simulink model "Snake_Robot_v1"  (R2022b)
settings: Solver=VariableStepAuto  StartTime=0.0  StopTime=300  RelTol=1e-5  AbsTol=1e-3  EnableMultiTasking=on
values from neighbouring files (symbols this model uses):
  amplitude = 2.5    [Snake_robot_parameters.m]
  frequency = 2    [Snake_robot_parameters.m]
  lookup_table_x = [-3 -1.5 -1 1 1.5 3]    [Snake_robot_parameters.m]
  lookup_table_y = [-3 -1.5 -1 1 1.5 3]    [Snake_robot_parameters.m]
  muk_x = 1e-5    (= 1e-05)    [Snake_robot_parameters.m]
  muk_y = 10    [Snake_robot_parameters.m]
  mus_x = 1e-4    (= 0.0001)    [Snake_robot_parameters.m]
  mus_y = 13    [Snake_robot_parameters.m]
  phase = 1.4    [Snake_robot_parameters.m]
undefined symbols (not defined in the file or in its folder): X, Y, Z
libraries: nesl_utility x88, sm_lib x74, simulink x53, slpidlib x5, robotalgslib x1
(part 3 of 4)

== system Snake_Robot_v1/body_1/custom friction law2 ==
  Demux : Demux  Outputs=2
  PS-Simulink Converter1 : nesl_utility/PS-Simulink Converter  PhysicalDomain=network_engine_domain  SubClassName=ps_output  LeftPortType=input  RightPortType=output  PseudoPeriodic=off  Frequencies=[]  VectorFormat=inherit  Unit=inherit  AffineConversion=off
  PS-Simulink Converter4 : nesl_utility/PS-Simulink Converter  PhysicalDomain=network_engine_domain  SubClassName=ps_output  LeftPortType=input  RightPortType=output  PseudoPeriodic=off  Frequencies=[]  VectorFormat=inherit  Unit=inherit  AffineConversion=off
  Scope{,1..3} (4 alike) : Scope
  Simulink-PS Converter : nesl_utility/Simulink-PS Converter  PhysicalDomain=network_engine_domain  SubClassName=ps_input  LeftPortType=input  RightPortType=output  PseudoPeriodic=off  Frequencies=[]  NoiseDistribution=none  NoiseParameters=[]  Unit=1  AffineConversion=off  FilteringAndDerivatives=provide  SimscapeFilterOrder=1  InputFilterTimeConstant=0.001  UdotUserProvided=0
  Spatial Contact Force : sm_lib/Forces and Torques/Spatial Contact Force  SenseContactBaseRotation=off  SenseContactBaseTranslation=off  CoefficientOfDynamicFriction=mu_dynamic  CoefficientOfStaticFriction=mu_static  NormalDamping=1e3  NormalDampingUnits=N/(m/s)  SenseContactSignal=off  NormalStiffness=1e6  NormalStiffnessUnits=N/m  FrictionalCriticalVelocity=1e-3  FrictionalCriticalVelocityUnits=m/s  ZeroCrossDetectContactStartAndEnd=off  SenseContactFollowerRotation=off  SenseContactFollowerTranslation=off  FrictionType=ProvidedByInput  SenseFrictionalForceMagnitude=off  SenseNormalForceMagnitude=on  NormalForceType=SmoothSpringDamper  SenseNormalVelocity=off  SenseSeparationDistance=off  SenseTangentialVelocity=on  NormalTransitionRegionWidth=1e-4  NormalTransitionRegionWidthUnits=m
  custom friction law : Subsystem
  body : PMIOPort  Side=Right
  ground : PMIOPort  Port=2  Side=Left
  wires:
  PS-Simulink Converter1/1 -> Demux/1, custom friction law/2(velocity)  "velocity"
  PS-Simulink Converter4/1 -> Scope1/1, custom friction law/1(normal force)  "normal force"
  custom friction law/1(Friction force) -> Scope/1, Simulink-PS Converter/1  "friction force"
  Demux/1 -> Scope2/1
  Demux/2 -> Scope3/1
  connections:
  Spatial Contact Force/LConn1 -- ground/RConn1
  Spatial Contact Force/RConn2 -- PS-Simulink Converter4/LConn1
  Simulink-PS Converter/RConn1 -- Spatial Contact Force/LConn2
  Spatial Contact Force/RConn3 -- PS-Simulink Converter1/LConn1
  Spatial Contact Force/RConn1 -- body/RConn1

== system Snake_Robot_v1/body_1/custom friction law3 ==
  Demux : Demux  Outputs=2
  PS-Simulink Converter1 : nesl_utility/PS-Simulink Converter  PhysicalDomain=network_engine_domain  SubClassName=ps_output  LeftPortType=input  RightPortType=output  PseudoPeriodic=off  Frequencies=[]  VectorFormat=inherit  Unit=inherit  AffineConversion=off
  PS-Simulink Converter4 : nesl_utility/PS-Simulink Converter  PhysicalDomain=network_engine_domain  SubClassName=ps_output  LeftPortType=input  RightPortType=output  PseudoPeriodic=off  Frequencies=[]  VectorFormat=inherit  Unit=inherit  AffineConversion=off
  Scope{,1..3} (4 alike) : Scope
  Simulink-PS Converter : nesl_utility/Simulink-PS Converter  PhysicalDomain=network_engine_domain  SubClassName=ps_input  LeftPortType=input  RightPortType=output  PseudoPeriodic=off  Frequencies=[]  NoiseDistribution=none  NoiseParameters=[]  Unit=1  AffineConversion=off  FilteringAndDerivatives=provide  SimscapeFilterOrder=1  InputFilterTimeConstant=0.001  UdotUserProvided=0
  Spatial Contact Force : sm_lib/Forces and Torques/Spatial Contact Force  SenseContactBaseRotation=off  SenseContactBaseTranslation=off  CoefficientOfDynamicFriction=mu_dynamic  CoefficientOfStaticFriction=mu_static  NormalDamping=1e3  NormalDampingUnits=N/(m/s)  SenseContactSignal=off  NormalStiffness=1e6  NormalStiffnessUnits=N/m  FrictionalCriticalVelocity=1e-3  FrictionalCriticalVelocityUnits=m/s  ZeroCrossDetectContactStartAndEnd=off  SenseContactFollowerRotation=off  SenseContactFollowerTranslation=off  FrictionType=ProvidedByInput  SenseFrictionalForceMagnitude=off  SenseNormalForceMagnitude=on  NormalForceType=SmoothSpringDamper  SenseNormalVelocity=off  SenseSeparationDistance=off  SenseTangentialVelocity=on  NormalTransitionRegionWidth=1e-4  NormalTransitionRegionWidthUnits=m
  custom friction law : Subsystem
  body : PMIOPort  Side=Right
  ground : PMIOPort  Port=2  Side=Left
  wires:
  Demux/2 -> Scope3/1
  Demux/1 -> Scope2/1
  custom friction law/1(Friction force) -> Simulink-PS Converter/1, Scope/1  "friction force"
  PS-Simulink Converter4/1 -> custom friction law/1(normal force), Scope1/1  "normal force"
  PS-Simulink Converter1/1 -> custom friction law/2(velocity), Demux/1  "velocity"
  connections:
  Spatial Contact Force/RConn1 -- body/RConn1
  Spatial Contact Force/RConn3 -- PS-Simulink Converter1/LConn1
  Simulink-PS Converter/RConn1 -- Spatial Contact Force/LConn2
  Spatial Contact Force/RConn2 -- PS-Simulink Converter4/LConn1
  Spatial Contact Force/LConn1 -- ground/RConn1

== system Snake_Robot_v1/body_2/custom friction law ==
  Demux : Demux  Outputs=2
  PS-Simulink Converter1 : nesl_utility/PS-Simulink Converter  PhysicalDomain=network_engine_domain  SubClassName=ps_output  LeftPortType=input  RightPortType=output  PseudoPeriodic=off  Frequencies=[]  VectorFormat=inherit  Unit=inherit  AffineConversion=off
  PS-Simulink Converter4 : nesl_utility/PS-Simulink Converter  PhysicalDomain=network_engine_domain  SubClassName=ps_output  LeftPortType=input  RightPortType=output  PseudoPeriodic=off  Frequencies=[]  VectorFormat=inherit  Unit=inherit  AffineConversion=off
  Scope{,1..3} (4 alike) : Scope
  Simulink-PS Converter : nesl_utility/Simulink-PS Converter  PhysicalDomain=network_engine_domain  SubClassName=ps_input  LeftPortType=input  RightPortType=output  PseudoPeriodic=off  Frequencies=[]  NoiseDistribution=none  NoiseParameters=[]  Unit=1  AffineConversion=off  FilteringAndDerivatives=provide  SimscapeFilterOrder=1  InputFilterTimeConstant=0.001  UdotUserProvided=0
  Spatial Contact Force : sm_lib/Forces and Torques/Spatial Contact Force  SenseContactBaseRotation=off  SenseContactBaseTranslation=off  CoefficientOfDynamicFriction=mu_dynamic  CoefficientOfStaticFriction=mu_static  NormalDamping=1e3  NormalDampingUnits=N/(m/s)  SenseContactSignal=off  NormalStiffness=1e6  NormalStiffnessUnits=N/m  FrictionalCriticalVelocity=1e-3  FrictionalCriticalVelocityUnits=m/s  ZeroCrossDetectContactStartAndEnd=off  SenseContactFollowerRotation=off  SenseContactFollowerTranslation=off  FrictionType=ProvidedByInput  SenseFrictionalForceMagnitude=off  SenseNormalForceMagnitude=on  NormalForceType=SmoothSpringDamper  SenseNormalVelocity=off  SenseSeparationDistance=off  SenseTangentialVelocity=on  NormalTransitionRegionWidth=1e-4  NormalTransitionRegionWidthUnits=m
  custom friction law : Subsystem
  body : PMIOPort  Side=Right
  ground : PMIOPort  Port=2  Side=Left
  wires:
  Demux/2 -> Scope3/1
  Demux/1 -> Scope2/1
  custom friction law/1(Friction force) -> Simulink-PS Converter/1, Scope/1  "friction force"
  PS-Simulink Converter4/1 -> custom friction law/1(normal force), Scope1/1  "normal force"
  PS-Simulink Converter1/1 -> custom friction law/2(velocity), Demux/1  "velocity"
  connections:
  Spatial Contact Force/RConn1 -- body/RConn1
  Spatial Contact Force/RConn3 -- PS-Simulink Converter1/LConn1
  Simulink-PS Converter/RConn1 -- Spatial Contact Force/LConn2
  Spatial Contact Force/RConn2 -- PS-Simulink Converter4/LConn1
  Spatial Contact Force/LConn1 -- ground/RConn1

== system Snake_Robot_v1/body_2/custom friction law1 ==
  Demux : Demux  Outputs=2
  PS-Simulink Converter1 : nesl_utility/PS-Simulink Converter  PhysicalDomain=network_engine_domain  SubClassName=ps_output  LeftPortType=input  RightPortType=output  PseudoPeriodic=off  Frequencies=[]  VectorFormat=inherit  Unit=inherit  AffineConversion=off
  PS-Simulink Converter4 : nesl_utility/PS-Simulink Converter  PhysicalDomain=network_engine_domain  SubClassName=ps_output  LeftPortType=input  RightPortType=output  PseudoPeriodic=off  Frequencies=[]  VectorFormat=inherit  Unit=inherit  AffineConversion=off
  Scope{,1..3} (4 alike) : Scope
  Simulink-PS Converter : nesl_utility/Simulink-PS Converter  PhysicalDomain=network_engine_domain  SubClassName=ps_input  LeftPortType=input  RightPortType=output  PseudoPeriodic=off  Frequencies=[]  NoiseDistribution=none  NoiseParameters=[]  Unit=1  AffineConversion=off  FilteringAndDerivatives=provide  SimscapeFilterOrder=1  InputFilterTimeConstant=0.001  UdotUserProvided=0
  Spatial Contact Force : sm_lib/Forces and Torques/Spatial Contact Force  SenseContactBaseRotation=off  SenseContactBaseTranslation=off  CoefficientOfDynamicFriction=mu_dynamic  CoefficientOfStaticFriction=mu_static  NormalDamping=1e3  NormalDampingUnits=N/(m/s)  SenseContactSignal=off  NormalStiffness=1e6  NormalStiffnessUnits=N/m  FrictionalCriticalVelocity=1e-3  FrictionalCriticalVelocityUnits=m/s  ZeroCrossDetectContactStartAndEnd=off  SenseContactFollowerRotation=off  SenseContactFollowerTranslation=off  FrictionType=ProvidedByInput  SenseFrictionalForceMagnitude=off  SenseNormalForceMagnitude=on  NormalForceType=SmoothSpringDamper  SenseNormalVelocity=off  SenseSeparationDistance=off  SenseTangentialVelocity=on  NormalTransitionRegionWidth=1e-4  NormalTransitionRegionWidthUnits=m
  custom friction law : Subsystem
  body : PMIOPort  Side=Right
  ground : PMIOPort  Port=2  Side=Left
  wires:
  PS-Simulink Converter1/1 -> Demux/1, custom friction law/2(velocity)  "velocity"
  PS-Simulink Converter4/1 -> Scope1/1, custom friction law/1(normal force)  "normal force"
  custom friction law/1(Friction force) -> Scope/1, Simulink-PS Converter/1  "friction force"
  Demux/1 -> Scope2/1
  Demux/2 -> Scope3/1
  connections:
  Spatial Contact Force/LConn1 -- ground/RConn1
  Spatial Contact Force/RConn2 -- PS-Simulink Converter4/LConn1
  Simulink-PS Converter/RConn1 -- Spatial Contact Force/LConn2
  Spatial Contact Force/RConn3 -- PS-Simulink Converter1/LConn1
  Spatial Contact Force/RConn1 -- body/RConn1

== system Snake_Robot_v1/body_2/custom friction law2 ==
  Demux : Demux  Outputs=2
  PS-Simulink Converter1 : nesl_utility/PS-Simulink Converter  PhysicalDomain=network_engine_domain  SubClassName=ps_output  LeftPortType=input  RightPortType=output  PseudoPeriodic=off  Frequencies=[]  VectorFormat=inherit  Unit=inherit  AffineConversion=off
  PS-Simulink Converter4 : nesl_utility/PS-Simulink Converter  PhysicalDomain=network_engine_domain  SubClassName=ps_output  LeftPortType=input  RightPortType=output  PseudoPeriodic=off  Frequencies=[]  VectorFormat=inherit  Unit=inherit  AffineConversion=off
  Scope{,1..3} (4 alike) : Scope
  Simulink-PS Converter : nesl_utility/Simulink-PS Converter  PhysicalDomain=network_engine_domain  SubClassName=ps_input  LeftPortType=input  RightPortType=output  PseudoPeriodic=off  Frequencies=[]  NoiseDistribution=none  NoiseParameters=[]  Unit=1  AffineConversion=off  FilteringAndDerivatives=provide  SimscapeFilterOrder=1  InputFilterTimeConstant=0.001  UdotUserProvided=0
  Spatial Contact Force : sm_lib/Forces and Torques/Spatial Contact Force  SenseContactBaseRotation=off  SenseContactBaseTranslation=off  CoefficientOfDynamicFriction=mu_dynamic  CoefficientOfStaticFriction=mu_static  NormalDamping=1e3  NormalDampingUnits=N/(m/s)  SenseContactSignal=off  NormalStiffness=1e6  NormalStiffnessUnits=N/m  FrictionalCriticalVelocity=1e-3  FrictionalCriticalVelocityUnits=m/s  ZeroCrossDetectContactStartAndEnd=off  SenseContactFollowerRotation=off  SenseContactFollowerTranslation=off  FrictionType=ProvidedByInput  SenseFrictionalForceMagnitude=off  SenseNormalForceMagnitude=on  NormalForceType=SmoothSpringDamper  SenseNormalVelocity=off  SenseSeparationDistance=off  SenseTangentialVelocity=on  NormalTransitionRegionWidth=1e-4  NormalTransitionRegionWidthUnits=m
  custom friction law : Subsystem
  body : PMIOPort  Side=Right
  ground : PMIOPort  Port=2  Side=Left
  wires:
  Demux/2 -> Scope3/1
  Demux/1 -> Scope2/1
  custom friction law/1(Friction force) -> Simulink-PS Converter/1, Scope/1  "friction force"
  PS-Simulink Converter4/1 -> custom friction law/1(normal force), Scope1/1  "normal force"
  PS-Simulink Converter1/1 -> custom friction law/2(velocity), Demux/1  "velocity"
  connections:
  Spatial Contact Force/RConn1 -- body/RConn1
  Spatial Contact Force/RConn3 -- PS-Simulink Converter1/LConn1
  Simulink-PS Converter/RConn1 -- Spatial Contact Force/LConn2
  Spatial Contact Force/RConn2 -- PS-Simulink Converter4/LConn1
  Spatial Contact Force/LConn1 -- ground/RConn1

== system Snake_Robot_v1/body_2/custom friction law3 ==
  Demux : Demux  Outputs=2
  PS-Simulink Converter1 : nesl_utility/PS-Simulink Converter  PhysicalDomain=network_engine_domain  SubClassName=ps_output  LeftPortType=input  RightPortType=output  PseudoPeriodic=off  Frequencies=[]  VectorFormat=inherit  Unit=inherit  AffineConversion=off
  PS-Simulink Converter4 : nesl_utility/PS-Simulink Converter  PhysicalDomain=network_engine_domain  SubClassName=ps_output  LeftPortType=input  RightPortType=output  PseudoPeriodic=off  Frequencies=[]  VectorFormat=inherit  Unit=inherit  AffineConversion=off
  Scope{,1..3} (4 alike) : Scope
  Simulink-PS Converter : nesl_utility/Simulink-PS Converter  PhysicalDomain=network_engine_domain  SubClassName=ps_input  LeftPortType=input  RightPortType=output  PseudoPeriodic=off  Frequencies=[]  NoiseDistribution=none  NoiseParameters=[]  Unit=1  AffineConversion=off  FilteringAndDerivatives=provide  SimscapeFilterOrder=1  InputFilterTimeConstant=0.001  UdotUserProvided=0
  Spatial Contact Force : sm_lib/Forces and Torques/Spatial Contact Force  SenseContactBaseRotation=off  SenseContactBaseTranslation=off  CoefficientOfDynamicFriction=mu_dynamic  CoefficientOfStaticFriction=mu_static  NormalDamping=1e3  NormalDampingUnits=N/(m/s)  SenseContactSignal=off  NormalStiffness=1e6  NormalStiffnessUnits=N/m  FrictionalCriticalVelocity=1e-3  FrictionalCriticalVelocityUnits=m/s  ZeroCrossDetectContactStartAndEnd=off  SenseContactFollowerRotation=off  SenseContactFollowerTranslation=off  FrictionType=ProvidedByInput  SenseFrictionalForceMagnitude=off  SenseNormalForceMagnitude=on  NormalForceType=SmoothSpringDamper  SenseNormalVelocity=off  SenseSeparationDistance=off  SenseTangentialVelocity=on  NormalTransitionRegionWidth=1e-4  NormalTransitionRegionWidthUnits=m
  custom friction law : Subsystem
  body : PMIOPort  Side=Right
  ground : PMIOPort  Port=2  Side=Left
  wires:
  PS-Simulink Converter1/1 -> Demux/1, custom friction law/2(velocity)  "velocity"
  PS-Simulink Converter4/1 -> Scope1/1, custom friction law/1(normal force)  "normal force"
  custom friction law/1(Friction force) -> Scope/1, Simulink-PS Converter/1  "friction force"
  Demux/1 -> Scope2/1
  Demux/2 -> Scope3/1
  connections:
  Spatial Contact Force/LConn1 -- ground/RConn1
  Spatial Contact Force/RConn2 -- PS-Simulink Converter4/LConn1
  Simulink-PS Converter/RConn1 -- Spatial Contact Force/LConn2
  Spatial Contact Force/RConn3 -- PS-Simulink Converter1/LConn1
  Spatial Contact Force/RConn1 -- body/RConn1

== system Snake_Robot_v1/body_3/custom friction law ==
  Demux : Demux  Outputs=2
  PS-Simulink Converter1 : nesl_utility/PS-Simulink Converter  PhysicalDomain=network_engine_domain  SubClassName=ps_output  LeftPortType=input  RightPortType=output  PseudoPeriodic=off  Frequencies=[]  VectorFormat=inherit  Unit=inherit  AffineConversion=off
  PS-Simulink Converter4 : nesl_utility/PS-Simulink Converter  PhysicalDomain=network_engine_domain  SubClassName=ps_output  LeftPortType=input  RightPortType=output  PseudoPeriodic=off  Frequencies=[]  VectorFormat=inherit  Unit=inherit  AffineConversion=off
  Scope{,1..3} (4 alike) : Scope
  Simulink-PS Converter : nesl_utility/Simulink-PS Converter  PhysicalDomain=network_engine_domain  SubClassName=ps_input  LeftPortType=input  RightPortType=output  PseudoPeriodic=off  Frequencies=[]  NoiseDistribution=none  NoiseParameters=[]  Unit=1  AffineConversion=off  FilteringAndDerivatives=provide  SimscapeFilterOrder=1  InputFilterTimeConstant=0.001  UdotUserProvided=0
  Spatial Contact Force : sm_lib/Forces and Torques/Spatial Contact Force  SenseContactBaseRotation=off  SenseContactBaseTranslation=off  CoefficientOfDynamicFriction=mu_dynamic  CoefficientOfStaticFriction=mu_static  NormalDamping=1e3  NormalDampingUnits=N/(m/s)  SenseContactSignal=off  NormalStiffness=1e6  NormalStiffnessUnits=N/m  FrictionalCriticalVelocity=1e-3  FrictionalCriticalVelocityUnits=m/s  ZeroCrossDetectContactStartAndEnd=off  SenseContactFollowerRotation=off  SenseContactFollowerTranslation=off  FrictionType=ProvidedByInput  SenseFrictionalForceMagnitude=off  SenseNormalForceMagnitude=on  NormalForceType=SmoothSpringDamper  SenseNormalVelocity=off  SenseSeparationDistance=off  SenseTangentialVelocity=on  NormalTransitionRegionWidth=1e-4  NormalTransitionRegionWidthUnits=m
  custom friction law : Subsystem
  body : PMIOPort  Side=Right
  ground : PMIOPort  Port=2  Side=Left
  wires:
  PS-Simulink Converter1/1 -> Demux/1, custom friction law/2(velocity)  "velocity"
  PS-Simulink Converter4/1 -> Scope1/1, custom friction law/1(normal force)  "normal force"
  custom friction law/1(Friction force) -> Scope/1, Simulink-PS Converter/1  "friction force"
  Demux/1 -> Scope2/1
  Demux/2 -> Scope3/1
  connections:
  Spatial Contact Force/LConn1 -- ground/RConn1
  Spatial Contact Force/RConn2 -- PS-Simulink Converter4/LConn1
  Simulink-PS Converter/RConn1 -- Spatial Contact Force/LConn2
  Spatial Contact Force/RConn3 -- PS-Simulink Converter1/LConn1
  Spatial Contact Force/RConn1 -- body/RConn1

== system Snake_Robot_v1/body_3/custom friction law1 ==
  Demux : Demux  Outputs=2
  PS-Simulink Converter1 : nesl_utility/PS-Simulink Converter  PhysicalDomain=network_engine_domain  SubClassName=ps_output  LeftPortType=input  RightPortType=output  PseudoPeriodic=off  Frequencies=[]  VectorFormat=inherit  Unit=inherit  AffineConversion=off
  PS-Simulink Converter4 : nesl_utility/PS-Simulink Converter  PhysicalDomain=network_engine_domain  SubClassName=ps_output  LeftPortType=input  RightPortType=output  PseudoPeriodic=off  Frequencies=[]  VectorFormat=inherit  Unit=inherit  AffineConversion=off
  Scope{,1..3} (4 alike) : Scope
  Simulink-PS Converter : nesl_utility/Simulink-PS Converter  PhysicalDomain=network_engine_domain  SubClassName=ps_input  LeftPortType=input  RightPortType=output  PseudoPeriodic=off  Frequencies=[]  NoiseDistribution=none  NoiseParameters=[]  Unit=1  AffineConversion=off  FilteringAndDerivatives=provide  SimscapeFilterOrder=1  InputFilterTimeConstant=0.001  UdotUserProvided=0
  Spatial Contact Force : sm_lib/Forces and Torques/Spatial Contact Force  SenseContactBaseRotation=off  SenseContactBaseTranslation=off  CoefficientOfDynamicFriction=mu_dynamic  CoefficientOfStaticFriction=mu_static  NormalDamping=1e3  NormalDampingUnits=N/(m/s)  SenseContactSignal=off  NormalStiffness=1e6  NormalStiffnessUnits=N/m  FrictionalCriticalVelocity=1e-3  FrictionalCriticalVelocityUnits=m/s  ZeroCrossDetectContactStartAndEnd=off  SenseContactFollowerRotation=off  SenseContactFollowerTranslation=off  FrictionType=ProvidedByInput  SenseFrictionalForceMagnitude=off  SenseNormalForceMagnitude=on  NormalForceType=SmoothSpringDamper  SenseNormalVelocity=off  SenseSeparationDistance=off  SenseTangentialVelocity=on  NormalTransitionRegionWidth=1e-4  NormalTransitionRegionWidthUnits=m
  custom friction law : Subsystem
  body : PMIOPort  Side=Right
  ground : PMIOPort  Port=2  Side=Left
  wires:
  Demux/2 -> Scope3/1
  Demux/1 -> Scope2/1
  custom friction law/1(Friction force) -> Simulink-PS Converter/1, Scope/1  "friction force"
  PS-Simulink Converter4/1 -> custom friction law/1(normal force), Scope1/1  "normal force"
  PS-Simulink Converter1/1 -> custom friction law/2(velocity), Demux/1  "velocity"
  connections:
  Spatial Contact Force/RConn1 -- body/RConn1
  Spatial Contact Force/RConn3 -- PS-Simulink Converter1/LConn1
  Simulink-PS Converter/RConn1 -- Spatial Contact Force/LConn2
  Spatial Contact Force/RConn2 -- PS-Simulink Converter4/LConn1
  Spatial Contact Force/LConn1 -- ground/RConn1

== system Snake_Robot_v1/body_3/custom friction law2 ==
  Demux : Demux  Outputs=2
  PS-Simulink Converter1 : nesl_utility/PS-Simulink Converter  PhysicalDomain=network_engine_domain  SubClassName=ps_output  LeftPortType=input  RightPortType=output  PseudoPeriodic=off  Frequencies=[]  VectorFormat=inherit  Unit=inherit  AffineConversion=off
  PS-Simulink Converter4 : nesl_utility/PS-Simulink Converter  PhysicalDomain=network_engine_domain  SubClassName=ps_output  LeftPortType=input  RightPortType=output  PseudoPeriodic=off  Frequencies=[]  VectorFormat=inherit  Unit=inherit  AffineConversion=off
  Scope{,1..3} (4 alike) : Scope
  Simulink-PS Converter : nesl_utility/Simulink-PS Converter  PhysicalDomain=network_engine_domain  SubClassName=ps_input  LeftPortType=input  RightPortType=output  PseudoPeriodic=off  Frequencies=[]  NoiseDistribution=none  NoiseParameters=[]  Unit=1  AffineConversion=off  FilteringAndDerivatives=provide  SimscapeFilterOrder=1  InputFilterTimeConstant=0.001  UdotUserProvided=0
  Spatial Contact Force : sm_lib/Forces and Torques/Spatial Contact Force  SenseContactBaseRotation=off  SenseContactBaseTranslation=off  CoefficientOfDynamicFriction=mu_dynamic  CoefficientOfStaticFriction=mu_static  NormalDamping=1e3  NormalDampingUnits=N/(m/s)  SenseContactSignal=off  NormalStiffness=1e6  NormalStiffnessUnits=N/m  FrictionalCriticalVelocity=1e-3  FrictionalCriticalVelocityUnits=m/s  ZeroCrossDetectContactStartAndEnd=off  SenseContactFollowerRotation=off  SenseContactFollowerTranslation=off  FrictionType=ProvidedByInput  SenseFrictionalForceMagnitude=off  SenseNormalForceMagnitude=on  NormalForceType=SmoothSpringDamper  SenseNormalVelocity=off  SenseSeparationDistance=off  SenseTangentialVelocity=on  NormalTransitionRegionWidth=1e-4  NormalTransitionRegionWidthUnits=m
  custom friction law : Subsystem
  body : PMIOPort  Side=Right
  ground : PMIOPort  Port=2  Side=Left
  wires:
  PS-Simulink Converter1/1 -> Demux/1, custom friction law/2(velocity)  "velocity"
  PS-Simulink Converter4/1 -> Scope1/1, custom friction law/1(normal force)  "normal force"
  custom friction law/1(Friction force) -> Scope/1, Simulink-PS Converter/1  "friction force"
  Demux/1 -> Scope2/1
  Demux/2 -> Scope3/1
  connections:
  Spatial Contact Force/LConn1 -- ground/RConn1
  Spatial Contact Force/RConn2 -- PS-Simulink Converter4/LConn1
  Simulink-PS Converter/RConn1 -- Spatial Contact Force/LConn2
  Spatial Contact Force/RConn3 -- PS-Simulink Converter1/LConn1
  Spatial Contact Force/RConn1 -- body/RConn1

== system Snake_Robot_v1/body_3/custom friction law3 ==
  Demux : Demux  Outputs=2
  PS-Simulink Converter1 : nesl_utility/PS-Simulink Converter  PhysicalDomain=network_engine_domain  SubClassName=ps_output  LeftPortType=input  RightPortType=output  PseudoPeriodic=off  Frequencies=[]  VectorFormat=inherit  Unit=inherit  AffineConversion=off
  PS-Simulink Converter4 : nesl_utility/PS-Simulink Converter  PhysicalDomain=network_engine_domain  SubClassName=ps_output  LeftPortType=input  RightPortType=output  PseudoPeriodic=off  Frequencies=[]  VectorFormat=inherit  Unit=inherit  AffineConversion=off
  Scope{,1..3} (4 alike) : Scope
  Simulink-PS Converter : nesl_utility/Simulink-PS Converter  PhysicalDomain=network_engine_domain  SubClassName=ps_input  LeftPortType=input  RightPortType=output  PseudoPeriodic=off  Frequencies=[]  NoiseDistribution=none  NoiseParameters=[]  Unit=1  AffineConversion=off  FilteringAndDerivatives=provide  SimscapeFilterOrder=1  InputFilterTimeConstant=0.001  UdotUserProvided=0
  Spatial Contact Force : sm_lib/Forces and Torques/Spatial Contact Force  SenseContactBaseRotation=off  SenseContactBaseTranslation=off  CoefficientOfDynamicFriction=mu_dynamic  CoefficientOfStaticFriction=mu_static  NormalDamping=1e3  NormalDampingUnits=N/(m/s)  SenseContactSignal=off  NormalStiffness=1e6  NormalStiffnessUnits=N/m  FrictionalCriticalVelocity=1e-3  FrictionalCriticalVelocityUnits=m/s  ZeroCrossDetectContactStartAndEnd=off  SenseContactFollowerRotation=off  SenseContactFollowerTranslation=off  FrictionType=ProvidedByInput  SenseFrictionalForceMagnitude=off  SenseNormalForceMagnitude=on  NormalForceType=SmoothSpringDamper  SenseNormalVelocity=off  SenseSeparationDistance=off  SenseTangentialVelocity=on  NormalTransitionRegionWidth=1e-4  NormalTransitionRegionWidthUnits=m
  custom friction law : Subsystem
  body : PMIOPort  Side=Right
  ground : PMIOPort  Port=2  Side=Left
  wires:
  Demux/2 -> Scope3/1
  Demux/1 -> Scope2/1
  custom friction law/1(Friction force) -> Simulink-PS Converter/1, Scope/1  "friction force"
  PS-Simulink Converter4/1 -> custom friction law/1(normal force), Scope1/1  "normal force"
  PS-Simulink Converter1/1 -> custom friction law/2(velocity), Demux/1  "velocity"
  connections:
  Spatial Contact Force/RConn1 -- body/RConn1
  Spatial Contact Force/RConn3 -- PS-Simulink Converter1/LConn1
  Simulink-PS Converter/RConn1 -- Spatial Contact Force/LConn2
  Spatial Contact Force/RConn2 -- PS-Simulink Converter4/LConn1
  Spatial Contact Force/LConn1 -- ground/RConn1

== system Snake_Robot_v1/body_4/custom friction law ==
  Demux : Demux  Outputs=2
  PS-Simulink Converter1 : nesl_utility/PS-Simulink Converter  PhysicalDomain=network_engine_domain  SubClassName=ps_output  LeftPortType=input  RightPortType=output  PseudoPeriodic=off  Frequencies=[]  VectorFormat=inherit  Unit=inherit  AffineConversion=off
  PS-Simulink Converter4 : nesl_utility/PS-Simulink Converter  PhysicalDomain=network_engine_domain  SubClassName=ps_output  LeftPortType=input  RightPortType=output  PseudoPeriodic=off  Frequencies=[]  VectorFormat=inherit  Unit=inherit  AffineConversion=off
  Scope{,1..3} (4 alike) : Scope
  Simulink-PS Converter : nesl_utility/Simulink-PS Converter  PhysicalDomain=network_engine_domain  SubClassName=ps_input  LeftPortType=input  RightPortType=output  PseudoPeriodic=off  Frequencies=[]  NoiseDistribution=none  NoiseParameters=[]  Unit=1  AffineConversion=off  FilteringAndDerivatives=provide  SimscapeFilterOrder=1  InputFilterTimeConstant=0.001  UdotUserProvided=0
  Spatial Contact Force : sm_lib/Forces and Torques/Spatial Contact Force  SenseContactBaseRotation=off  SenseContactBaseTranslation=off  CoefficientOfDynamicFriction=mu_dynamic  CoefficientOfStaticFriction=mu_static  NormalDamping=1e3  NormalDampingUnits=N/(m/s)  SenseContactSignal=off  NormalStiffness=1e6  NormalStiffnessUnits=N/m  FrictionalCriticalVelocity=1e-3  FrictionalCriticalVelocityUnits=m/s  ZeroCrossDetectContactStartAndEnd=off  SenseContactFollowerRotation=off  SenseContactFollowerTranslation=off  FrictionType=ProvidedByInput  SenseFrictionalForceMagnitude=off  SenseNormalForceMagnitude=on  NormalForceType=SmoothSpringDamper  SenseNormalVelocity=off  SenseSeparationDistance=off  SenseTangentialVelocity=on  NormalTransitionRegionWidth=1e-4  NormalTransitionRegionWidthUnits=m
  custom friction law : Subsystem
  body : PMIOPort  Side=Right
  ground : PMIOPort  Port=2  Side=Left
  wires:
  Demux/2 -> Scope3/1
  Demux/1 -> Scope2/1
  custom friction law/1(Friction force) -> Simulink-PS Converter/1, Scope/1  "friction force"
  PS-Simulink Converter4/1 -> custom friction law/1(normal force), Scope1/1  "normal force"
  PS-Simulink Converter1/1 -> custom friction law/2(velocity), Demux/1  "velocity"
  connections:
  Spatial Contact Force/RConn1 -- body/RConn1
  Spatial Contact Force/RConn3 -- PS-Simulink Converter1/LConn1
  Simulink-PS Converter/RConn1 -- Spatial Contact Force/LConn2
  Spatial Contact Force/RConn2 -- PS-Simulink Converter4/LConn1
  Spatial Contact Force/LConn1 -- ground/RConn1

== system Snake_Robot_v1/body_4/custom friction law1 ==
  Demux : Demux  Outputs=2
  PS-Simulink Converter1 : nesl_utility/PS-Simulink Converter  PhysicalDomain=network_engine_domain  SubClassName=ps_output  LeftPortType=input  RightPortType=output  PseudoPeriodic=off  Frequencies=[]  VectorFormat=inherit  Unit=inherit  AffineConversion=off
  PS-Simulink Converter4 : nesl_utility/PS-Simulink Converter  PhysicalDomain=network_engine_domain  SubClassName=ps_output  LeftPortType=input  RightPortType=output  PseudoPeriodic=off  Frequencies=[]  VectorFormat=inherit  Unit=inherit  AffineConversion=off
  Scope{,1..3} (4 alike) : Scope
  Simulink-PS Converter : nesl_utility/Simulink-PS Converter  PhysicalDomain=network_engine_domain  SubClassName=ps_input  LeftPortType=input  RightPortType=output  PseudoPeriodic=off  Frequencies=[]  NoiseDistribution=none  NoiseParameters=[]  Unit=1  AffineConversion=off  FilteringAndDerivatives=provide  SimscapeFilterOrder=1  InputFilterTimeConstant=0.001  UdotUserProvided=0
  Spatial Contact Force : sm_lib/Forces and Torques/Spatial Contact Force  SenseContactBaseRotation=off  SenseContactBaseTranslation=off  CoefficientOfDynamicFriction=mu_dynamic  CoefficientOfStaticFriction=mu_static  NormalDamping=1e3  NormalDampingUnits=N/(m/s)  SenseContactSignal=off  NormalStiffness=1e6  NormalStiffnessUnits=N/m  FrictionalCriticalVelocity=1e-3  FrictionalCriticalVelocityUnits=m/s  ZeroCrossDetectContactStartAndEnd=off  SenseContactFollowerRotation=off  SenseContactFollowerTranslation=off  FrictionType=ProvidedByInput  SenseFrictionalForceMagnitude=off  SenseNormalForceMagnitude=on  NormalForceType=SmoothSpringDamper  SenseNormalVelocity=off  SenseSeparationDistance=off  SenseTangentialVelocity=on  NormalTransitionRegionWidth=1e-4  NormalTransitionRegionWidthUnits=m
  custom friction law : Subsystem
  body : PMIOPort  Side=Right
  ground : PMIOPort  Port=2  Side=Left
  wires:
  PS-Simulink Converter1/1 -> Demux/1, custom friction law/2(velocity)  "velocity"
  PS-Simulink Converter4/1 -> Scope1/1, custom friction law/1(normal force)  "normal force"
  custom friction law/1(Friction force) -> Scope/1, Simulink-PS Converter/1  "friction force"
  Demux/1 -> Scope2/1
  Demux/2 -> Scope3/1
  connections:
  Spatial Contact Force/LConn1 -- ground/RConn1
  Spatial Contact Force/RConn2 -- PS-Simulink Converter4/LConn1
  Simulink-PS Converter/RConn1 -- Spatial Contact Force/LConn2
  Spatial Contact Force/RConn3 -- PS-Simulink Converter1/LConn1
  Spatial Contact Force/RConn1 -- body/RConn1

== system Snake_Robot_v1/body_4/custom friction law2 ==
  Demux : Demux  Outputs=2
  PS-Simulink Converter1 : nesl_utility/PS-Simulink Converter  PhysicalDomain=network_engine_domain  SubClassName=ps_output  LeftPortType=input  RightPortType=output  PseudoPeriodic=off  Frequencies=[]  VectorFormat=inherit  Unit=inherit  AffineConversion=off
  PS-Simulink Converter4 : nesl_utility/PS-Simulink Converter  PhysicalDomain=network_engine_domain  SubClassName=ps_output  LeftPortType=input  RightPortType=output  PseudoPeriodic=off  Frequencies=[]  VectorFormat=inherit  Unit=inherit  AffineConversion=off
  Scope{,1..3} (4 alike) : Scope
  Simulink-PS Converter : nesl_utility/Simulink-PS Converter  PhysicalDomain=network_engine_domain  SubClassName=ps_input  LeftPortType=input  RightPortType=output  PseudoPeriodic=off  Frequencies=[]  NoiseDistribution=none  NoiseParameters=[]  Unit=1  AffineConversion=off  FilteringAndDerivatives=provide  SimscapeFilterOrder=1  InputFilterTimeConstant=0.001  UdotUserProvided=0
  Spatial Contact Force : sm_lib/Forces and Torques/Spatial Contact Force  SenseContactBaseRotation=off  SenseContactBaseTranslation=off  CoefficientOfDynamicFriction=mu_dynamic  CoefficientOfStaticFriction=mu_static  NormalDamping=1e3  NormalDampingUnits=N/(m/s)  SenseContactSignal=off  NormalStiffness=1e6  NormalStiffnessUnits=N/m  FrictionalCriticalVelocity=1e-3  FrictionalCriticalVelocityUnits=m/s  ZeroCrossDetectContactStartAndEnd=off  SenseContactFollowerRotation=off  SenseContactFollowerTranslation=off  FrictionType=ProvidedByInput  SenseFrictionalForceMagnitude=off  SenseNormalForceMagnitude=on  NormalForceType=SmoothSpringDamper  SenseNormalVelocity=off  SenseSeparationDistance=off  SenseTangentialVelocity=on  NormalTransitionRegionWidth=1e-4  NormalTransitionRegionWidthUnits=m
  custom friction law : Subsystem
  body : PMIOPort  Side=Right
  ground : PMIOPort  Port=2  Side=Left
  wires:
  Demux/2 -> Scope3/1
  Demux/1 -> Scope2/1
  custom friction law/1(Friction force) -> Simulink-PS Converter/1, Scope/1  "friction force"
  PS-Simulink Converter4/1 -> custom friction law/1(normal force), Scope1/1  "normal force"
  PS-Simulink Converter1/1 -> custom friction law/2(velocity), Demux/1  "velocity"
  connections:
  Spatial Contact Force/RConn1 -- body/RConn1
  Spatial Contact Force/RConn3 -- PS-Simulink Converter1/LConn1
  Simulink-PS Converter/RConn1 -- Spatial Contact Force/LConn2
  Spatial Contact Force/RConn2 -- PS-Simulink Converter4/LConn1
  Spatial Contact Force/LConn1 -- ground/RConn1

== system Snake_Robot_v1/body_4/custom friction law3 ==
  Demux : Demux  Outputs=2
  PS-Simulink Converter1 : nesl_utility/PS-Simulink Converter  PhysicalDomain=network_engine_domain  SubClassName=ps_output  LeftPortType=input  RightPortType=output  PseudoPeriodic=off  Frequencies=[]  VectorFormat=inherit  Unit=inherit  AffineConversion=off
  PS-Simulink Converter4 : nesl_utility/PS-Simulink Converter  PhysicalDomain=network_engine_domain  SubClassName=ps_output  LeftPortType=input  RightPortType=output  PseudoPeriodic=off  Frequencies=[]  VectorFormat=inherit  Unit=inherit  AffineConversion=off
  Scope{,1..3} (4 alike) : Scope
  Simulink-PS Converter : nesl_utility/Simulink-PS Converter  PhysicalDomain=network_engine_domain  SubClassName=ps_input  LeftPortType=input  RightPortType=output  PseudoPeriodic=off  Frequencies=[]  NoiseDistribution=none  NoiseParameters=[]  Unit=1  AffineConversion=off  FilteringAndDerivatives=provide  SimscapeFilterOrder=1  InputFilterTimeConstant=0.001  UdotUserProvided=0
  Spatial Contact Force : sm_lib/Forces and Torques/Spatial Contact Force  SenseContactBaseRotation=off  SenseContactBaseTranslation=off  CoefficientOfDynamicFriction=mu_dynamic  CoefficientOfStaticFriction=mu_static  NormalDamping=1e3  NormalDampingUnits=N/(m/s)  SenseContactSignal=off  NormalStiffness=1e6  NormalStiffnessUnits=N/m  FrictionalCriticalVelocity=1e-3  FrictionalCriticalVelocityUnits=m/s  ZeroCrossDetectContactStartAndEnd=off  SenseContactFollowerRotation=off  SenseContactFollowerTranslation=off  FrictionType=ProvidedByInput  SenseFrictionalForceMagnitude=off  SenseNormalForceMagnitude=on  NormalForceType=SmoothSpringDamper  SenseNormalVelocity=off  SenseSeparationDistance=off  SenseTangentialVelocity=on  NormalTransitionRegionWidth=1e-4  NormalTransitionRegionWidthUnits=m
  custom friction law : Subsystem
  body : PMIOPort  Side=Right
  ground : PMIOPort  Port=2  Side=Left
  wires:
  PS-Simulink Converter1/1 -> Demux/1, custom friction law/2(velocity)  "velocity"
  PS-Simulink Converter4/1 -> Scope1/1, custom friction law/1(normal force)  "normal force"
  custom friction law/1(Friction force) -> Scope/1, Simulink-PS Converter/1  "friction force"
  Demux/1 -> Scope2/1
  Demux/2 -> Scope3/1
  connections:
  Spatial Contact Force/LConn1 -- ground/RConn1
  Spatial Contact Force/RConn2 -- PS-Simulink Converter4/LConn1
  Simulink-PS Converter/RConn1 -- Spatial Contact Force/LConn2
  Spatial Contact Force/RConn3 -- PS-Simulink Converter1/LConn1
  Spatial Contact Force/RConn1 -- body/RConn1

== system Snake_Robot_v1/body_5/custom friction law ==
  Demux : Demux  Outputs=2
  PS-Simulink Converter1 : nesl_utility/PS-Simulink Converter  PhysicalDomain=network_engine_domain  SubClassName=ps_output  LeftPortType=input  RightPortType=output  PseudoPeriodic=off  Frequencies=[]  VectorFormat=inherit  Unit=inherit  AffineConversion=off
  PS-Simulink Converter4 : nesl_utility/PS-Simulink Converter  PhysicalDomain=network_engine_domain  SubClassName=ps_output  LeftPortType=input  RightPortType=output  PseudoPeriodic=off  Frequencies=[]  VectorFormat=inherit  Unit=inherit  AffineConversion=off
  Scope{,1..3} (4 alike) : Scope
  Simulink-PS Converter : nesl_utility/Simulink-PS Converter  PhysicalDomain=network_engine_domain  SubClassName=ps_input  LeftPortType=input  RightPortType=output  PseudoPeriodic=off  Frequencies=[]  NoiseDistribution=none  NoiseParameters=[]  Unit=1  AffineConversion=off  FilteringAndDerivatives=provide  SimscapeFilterOrder=1  InputFilterTimeConstant=0.001  UdotUserProvided=0
  Spatial Contact Force : sm_lib/Forces and Torques/Spatial Contact Force  SenseContactBaseRotation=off  SenseContactBaseTranslation=off  CoefficientOfDynamicFriction=mu_dynamic  CoefficientOfStaticFriction=mu_static  NormalDamping=1e3  NormalDampingUnits=N/(m/s)  SenseContactSignal=off  NormalStiffness=1e6  NormalStiffnessUnits=N/m  FrictionalCriticalVelocity=1e-3  FrictionalCriticalVelocityUnits=m/s  ZeroCrossDetectContactStartAndEnd=off  SenseContactFollowerRotation=off  SenseContactFollowerTranslation=off  FrictionType=ProvidedByInput  SenseFrictionalForceMagnitude=off  SenseNormalForceMagnitude=on  NormalForceType=SmoothSpringDamper  SenseNormalVelocity=off  SenseSeparationDistance=off  SenseTangentialVelocity=on  NormalTransitionRegionWidth=1e-4  NormalTransitionRegionWidthUnits=m
  custom friction law : Subsystem
  body : PMIOPort  Side=Right
  ground : PMIOPort  Port=2  Side=Left
  wires:
  PS-Simulink Converter1/1 -> Demux/1, custom friction law/2(velocity)  "velocity"
  PS-Simulink Converter4/1 -> Scope1/1, custom friction law/1(normal force)  "normal force"
  custom friction law/1(Friction force) -> Scope/1, Simulink-PS Converter/1  "friction force"
  Demux/1 -> Scope2/1
  Demux/2 -> Scope3/1
  connections:
  Spatial Contact Force/LConn1 -- ground/RConn1
  Spatial Contact Force/RConn2 -- PS-Simulink Converter4/LConn1
  Simulink-PS Converter/RConn1 -- Spatial Contact Force/LConn2
  Spatial Contact Force/RConn3 -- PS-Simulink Converter1/LConn1
  Spatial Contact Force/RConn1 -- body/RConn1

== system Snake_Robot_v1/body_5/custom friction law1 ==
  Demux : Demux  Outputs=2
  PS-Simulink Converter1 : nesl_utility/PS-Simulink Converter  PhysicalDomain=network_engine_domain  SubClassName=ps_output  LeftPortType=input  RightPortType=output  PseudoPeriodic=off  Frequencies=[]  VectorFormat=inherit  Unit=inherit  AffineConversion=off
  PS-Simulink Converter4 : nesl_utility/PS-Simulink Converter  PhysicalDomain=network_engine_domain  SubClassName=ps_output  LeftPortType=input  RightPortType=output  PseudoPeriodic=off  Frequencies=[]  VectorFormat=inherit  Unit=inherit  AffineConversion=off
  Scope{,1..3} (4 alike) : Scope
  Simulink-PS Converter : nesl_utility/Simulink-PS Converter  PhysicalDomain=network_engine_domain  SubClassName=ps_input  LeftPortType=input  RightPortType=output  PseudoPeriodic=off  Frequencies=[]  NoiseDistribution=none  NoiseParameters=[]  Unit=1  AffineConversion=off  FilteringAndDerivatives=provide  SimscapeFilterOrder=1  InputFilterTimeConstant=0.001  UdotUserProvided=0
  Spatial Contact Force : sm_lib/Forces and Torques/Spatial Contact Force  SenseContactBaseRotation=off  SenseContactBaseTranslation=off  CoefficientOfDynamicFriction=mu_dynamic  CoefficientOfStaticFriction=mu_static  NormalDamping=1e3  NormalDampingUnits=N/(m/s)  SenseContactSignal=off  NormalStiffness=1e6  NormalStiffnessUnits=N/m  FrictionalCriticalVelocity=1e-3  FrictionalCriticalVelocityUnits=m/s  ZeroCrossDetectContactStartAndEnd=off  SenseContactFollowerRotation=off  SenseContactFollowerTranslation=off  FrictionType=ProvidedByInput  SenseFrictionalForceMagnitude=off  SenseNormalForceMagnitude=on  NormalForceType=SmoothSpringDamper  SenseNormalVelocity=off  SenseSeparationDistance=off  SenseTangentialVelocity=on  NormalTransitionRegionWidth=1e-4  NormalTransitionRegionWidthUnits=m
  custom friction law : Subsystem
  body : PMIOPort  Side=Right
  ground : PMIOPort  Port=2  Side=Left
  wires:
  Demux/2 -> Scope3/1
  Demux/1 -> Scope2/1
  custom friction law/1(Friction force) -> Simulink-PS Converter/1, Scope/1  "friction force"
  PS-Simulink Converter4/1 -> custom friction law/1(normal force), Scope1/1  "normal force"
  PS-Simulink Converter1/1 -> custom friction law/2(velocity), Demux/1  "velocity"
  connections:
  Spatial Contact Force/RConn1 -- body/RConn1
  Spatial Contact Force/RConn3 -- PS-Simulink Converter1/LConn1
  Simulink-PS Converter/RConn1 -- Spatial Contact Force/LConn2
  Spatial Contact Force/RConn2 -- PS-Simulink Converter4/LConn1
  Spatial Contact Force/LConn1 -- ground/RConn1

== system Snake_Robot_v1/body_5/custom friction law2 ==
  Demux : Demux  Outputs=2
  PS-Simulink Converter1 : nesl_utility/PS-Simulink Converter  PhysicalDomain=network_engine_domain  SubClassName=ps_output  LeftPortType=input  RightPortType=output  PseudoPeriodic=off  Frequencies=[]  VectorFormat=inherit  Unit=inherit  AffineConversion=off
  PS-Simulink Converter4 : nesl_utility/PS-Simulink Converter  PhysicalDomain=network_engine_domain  SubClassName=ps_output  LeftPortType=input  RightPortType=output  PseudoPeriodic=off  Frequencies=[]  VectorFormat=inherit  Unit=inherit  AffineConversion=off
  Scope{,1..3} (4 alike) : Scope
  Simulink-PS Converter : nesl_utility/Simulink-PS Converter  PhysicalDomain=network_engine_domain  SubClassName=ps_input  LeftPortType=input  RightPortType=output  PseudoPeriodic=off  Frequencies=[]  NoiseDistribution=none  NoiseParameters=[]  Unit=1  AffineConversion=off  FilteringAndDerivatives=provide  SimscapeFilterOrder=1  InputFilterTimeConstant=0.001  UdotUserProvided=0
  Spatial Contact Force : sm_lib/Forces and Torques/Spatial Contact Force  SenseContactBaseRotation=off  SenseContactBaseTranslation=off  CoefficientOfDynamicFriction=mu_dynamic  CoefficientOfStaticFriction=mu_static  NormalDamping=1e3  NormalDampingUnits=N/(m/s)  SenseContactSignal=off  NormalStiffness=1e6  NormalStiffnessUnits=N/m  FrictionalCriticalVelocity=1e-3  FrictionalCriticalVelocityUnits=m/s  ZeroCrossDetectContactStartAndEnd=off  SenseContactFollowerRotation=off  SenseContactFollowerTranslation=off  FrictionType=ProvidedByInput  SenseFrictionalForceMagnitude=off  SenseNormalForceMagnitude=on  NormalForceType=SmoothSpringDamper  SenseNormalVelocity=off  SenseSeparationDistance=off  SenseTangentialVelocity=on  NormalTransitionRegionWidth=1e-4  NormalTransitionRegionWidthUnits=m
  custom friction law : Subsystem
  body : PMIOPort  Side=Right
  ground : PMIOPort  Port=2  Side=Left
  wires:
  PS-Simulink Converter1/1 -> Demux/1, custom friction law/2(velocity)  "velocity"
  PS-Simulink Converter4/1 -> Scope1/1, custom friction law/1(normal force)  "normal force"
  custom friction law/1(Friction force) -> Scope/1, Simulink-PS Converter/1  "friction force"
  Demux/1 -> Scope2/1
  Demux/2 -> Scope3/1
  connections:
  Spatial Contact Force/LConn1 -- ground/RConn1
  Spatial Contact Force/RConn2 -- PS-Simulink Converter4/LConn1
  Simulink-PS Converter/RConn1 -- Spatial Contact Force/LConn2
  Spatial Contact Force/RConn3 -- PS-Simulink Converter1/LConn1
  Spatial Contact Force/RConn1 -- body/RConn1

== system Snake_Robot_v1/body_5/custom friction law3 ==
  Demux : Demux  Outputs=2
  PS-Simulink Converter1 : nesl_utility/PS-Simulink Converter  PhysicalDomain=network_engine_domain  SubClassName=ps_output  LeftPortType=input  RightPortType=output  PseudoPeriodic=off  Frequencies=[]  VectorFormat=inherit  Unit=inherit  AffineConversion=off
  PS-Simulink Converter4 : nesl_utility/PS-Simulink Converter  PhysicalDomain=network_engine_domain  SubClassName=ps_output  LeftPortType=input  RightPortType=output  PseudoPeriodic=off  Frequencies=[]  VectorFormat=inherit  Unit=inherit  AffineConversion=off
  Scope{,1..3} (4 alike) : Scope
  Simulink-PS Converter : nesl_utility/Simulink-PS Converter  PhysicalDomain=network_engine_domain  SubClassName=ps_input  LeftPortType=input  RightPortType=output  PseudoPeriodic=off  Frequencies=[]  NoiseDistribution=none  NoiseParameters=[]  Unit=1  AffineConversion=off  FilteringAndDerivatives=provide  SimscapeFilterOrder=1  InputFilterTimeConstant=0.001  UdotUserProvided=0
  Spatial Contact Force : sm_lib/Forces and Torques/Spatial Contact Force  SenseContactBaseRotation=off  SenseContactBaseTranslation=off  CoefficientOfDynamicFriction=mu_dynamic  CoefficientOfStaticFriction=mu_static  NormalDamping=1e3  NormalDampingUnits=N/(m/s)  SenseContactSignal=off  NormalStiffness=1e6  NormalStiffnessUnits=N/m  FrictionalCriticalVelocity=1e-3  FrictionalCriticalVelocityUnits=m/s  ZeroCrossDetectContactStartAndEnd=off  SenseContactFollowerRotation=off  SenseContactFollowerTranslation=off  FrictionType=ProvidedByInput  SenseFrictionalForceMagnitude=off  SenseNormalForceMagnitude=on  NormalForceType=SmoothSpringDamper  SenseNormalVelocity=off  SenseSeparationDistance=off  SenseTangentialVelocity=on  NormalTransitionRegionWidth=1e-4  NormalTransitionRegionWidthUnits=m
  custom friction law : Subsystem
  body : PMIOPort  Side=Right
  ground : PMIOPort  Port=2  Side=Left
  wires:
  Demux/2 -> Scope3/1
  Demux/1 -> Scope2/1
  custom friction law/1(Friction force) -> Simulink-PS Converter/1, Scope/1  "friction force"
  PS-Simulink Converter4/1 -> custom friction law/1(normal force), Scope1/1  "normal force"
  PS-Simulink Converter1/1 -> custom friction law/2(velocity), Demux/1  "velocity"
  connections:
  Spatial Contact Force/RConn1 -- body/RConn1
  Spatial Contact Force/RConn3 -- PS-Simulink Converter1/LConn1
  Simulink-PS Converter/RConn1 -- Spatial Contact Force/LConn2
  Spatial Contact Force/RConn2 -- PS-Simulink Converter4/LConn1
  Spatial Contact Force/LConn1 -- ground/RConn1

== system Snake_Robot_v1/body_6/custom friction law ==
  Demux : Demux  Outputs=2
  PS-Simulink Converter1 : nesl_utility/PS-Simulink Converter  PhysicalDomain=network_engine_domain  SubClassName=ps_output  LeftPortType=input  RightPortType=output  PseudoPeriodic=off  Frequencies=[]  VectorFormat=inherit  Unit=inherit  AffineConversion=off
  PS-Simulink Converter4 : nesl_utility/PS-Simulink Converter  PhysicalDomain=network_engine_domain  SubClassName=ps_output  LeftPortType=input  RightPortType=output  PseudoPeriodic=off  Frequencies=[]  VectorFormat=inherit  Unit=inherit  AffineConversion=off
  Scope{,1..3} (4 alike) : Scope
  Simulink-PS Converter : nesl_utility/Simulink-PS Converter  PhysicalDomain=network_engine_domain  SubClassName=ps_input  LeftPortType=input  RightPortType=output  PseudoPeriodic=off  Frequencies=[]  NoiseDistribution=none  NoiseParameters=[]  Unit=1  AffineConversion=off  FilteringAndDerivatives=provide  SimscapeFilterOrder=1  InputFilterTimeConstant=0.001  UdotUserProvided=0
  Spatial Contact Force : sm_lib/Forces and Torques/Spatial Contact Force  SenseContactBaseRotation=off  SenseContactBaseTranslation=off  CoefficientOfDynamicFriction=mu_dynamic  CoefficientOfStaticFriction=mu_static  NormalDamping=1e3  NormalDampingUnits=N/(m/s)  SenseContactSignal=off  NormalStiffness=1e6  NormalStiffnessUnits=N/m  FrictionalCriticalVelocity=1e-3  FrictionalCriticalVelocityUnits=m/s  ZeroCrossDetectContactStartAndEnd=off  SenseContactFollowerRotation=off  SenseContactFollowerTranslation=off  FrictionType=ProvidedByInput  SenseFrictionalForceMagnitude=off  SenseNormalForceMagnitude=on  NormalForceType=SmoothSpringDamper  SenseNormalVelocity=off  SenseSeparationDistance=off  SenseTangentialVelocity=on  NormalTransitionRegionWidth=1e-4  NormalTransitionRegionWidthUnits=m
  custom friction law : Subsystem
  body : PMIOPort  Side=Right
  ground : PMIOPort  Port=2  Side=Left
  wires:
  Demux/2 -> Scope3/1
  Demux/1 -> Scope2/1
  custom friction law/1(Friction force) -> Simulink-PS Converter/1, Scope/1  "friction force"
  PS-Simulink Converter4/1 -> custom friction law/1(normal force), Scope1/1  "normal force"
  PS-Simulink Converter1/1 -> custom friction law/2(velocity), Demux/1  "velocity"
  connections:
  Spatial Contact Force/RConn1 -- body/RConn1
  Spatial Contact Force/RConn3 -- PS-Simulink Converter1/LConn1
  Simulink-PS Converter/RConn1 -- Spatial Contact Force/LConn2
  Spatial Contact Force/RConn2 -- PS-Simulink Converter4/LConn1
  Spatial Contact Force/LConn1 -- ground/RConn1
